simulink library "vehdynlibtirecommon_TUM"  (R2018b)
settings: Solver=ode45  StartTime=0.0  StopTime=10.0  RelTol=1e-3  EnableMultiTasking=on
undefined symbols (not defined in the file): br, drum_a, drum_abore, drum_c, drum_r, drum_theta1, drum_theta2, g, IYY, mu_kinetic, mu_static, omegao, T_RelaxationMy, tireStruct, UNLOADED_RADIUS, zdoto, zo
libraries: autolibsharedcommon x2, autolibutils x1
Description:
  | Automotive Blockset Library: Components used in the Tire Dynamics Library
settings Model: ModifiedByFormat=The MathWorks, Inc.  Creator=The MathWorks, Inc.  LastModifiedBy=The MathWorks, Inc.
settings SolverCC: MinimalZcImpactIntegration=on
settings DataIOCC: LimitDataPoints=on  SaveFormat=Array
settings OptimizationCC: LifeSpan=inf
settings DebuggingCC: AllowSymbolicDim=off  LibraryContextMissingDiagnostic=none  SFUnexpectedBacktrackingDiag=warning  SFNoUnconditionalDefaultTransitionDiag=warning  SFExecutionAtInitializationDiag=none
settings HardwareCC: ProdBitPerPointer=32  ProdBitPerSizeT=32  ProdBitPerPtrDiffT=32  ProdLargestAtomicFloat=None  ProdIntDivRoundTo=Undefined  ProdEndianess=Unspecified  ProdWordSize=32  ProdHWDeviceType=32-bit Generic
settings ModelReferenceCC: PropagateSignalLabelsOutOfModel=off
settings SFSimCC: SimUseLocalCustomCode=off
settings RTWCC: RTWUseLocalCustomCode=off
settings CodeAppCC: StateflowObjectComments=on
settings GRTTargetCC: TargetLangStandard=C89/C90 (ANSI)  GeneratePreprocessorConditionals=Disable all
settings ConfigComp: CovMetricSettings=dw  CovHtmlReporting=on  CovSaveCumulativeToWorkspaceVar=on  CovSaveSingleToWorkspaceVar=on  CovShowResultsExplorer=off  CovExternalEMLEnable=off

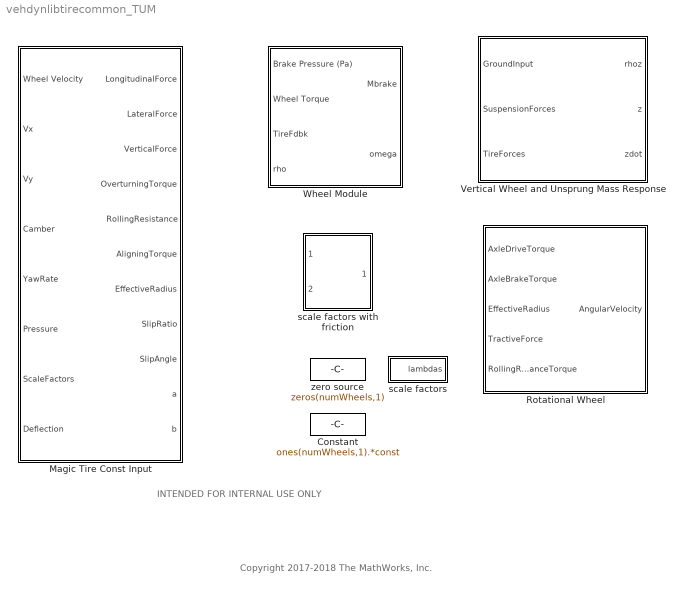
== system vehdynlibtirecommon_TUM ==
  note: INTENDED FOR INTERNAL USE ONLY
  note: Copyright 2017-2018 The MathWorks, Inc.
  Constant : Constant  Value=ones(numWheels,1).*const  mask{const=220000, numWheels=1}
      mask prompts: const "Constant Value"; numWheels "Number of wheels"
  Magic Tire Const Input : Subsystem
  Rotational Wheel : Subsystem  mask{Iyy=tireStruct(:).IYY, rhodot_o=omegao, br=br}
      mask prompts: Iyy "Wheel inertia [kg*m^2]"; rhodot_o "Initial wheel velocity [rad/s]"; br "Rotational damping [N*m*s/rad]"
  Vertical Wheel and Unsprung Mass Response : Subsystem  mask{m=tireStruct(:).MASS, bz=vertcat(tireStruct(:).VERTICAL_DAMPING), zo=zo, zdoto=zdoto, g=g, ReMax=.15}
      mask prompts: m "Unsprung mass [m]"; bz "Vertical damping [N*m/s]"; zo "Initial deflection [m]"; zdoto "Initial velocity [m/s]"; g "Gravitational acceleration [m/s^2]"; ReMax "Maximum unloaded radius [m]:"
  Wheel Module : Subsystem
  scale factors : Subsystem  mask{numWheels=1}
      mask prompts: numWheels "Number of wheels"
  scale factors with friction : Subsystem  mask{numWheels=1}
      mask prompts: numWheels "Number of wheels"
  zero source : Constant  Value=zeros(numWheels,1)  mask{numWheels=1}
      mask prompts: numWheels "Number of wheels"

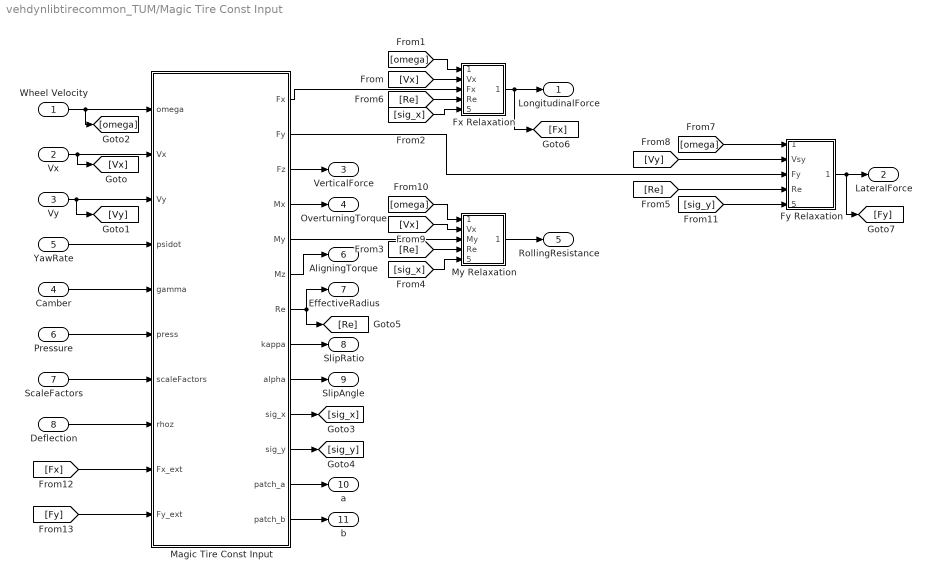
== system vehdynlibtirecommon_TUM/Magic Tire Const Input ==
  Wheel Velocity : Inport
  Vx : Inport  Port=2
  Vy : Inport  Port=3
  Camber : Inport  Port=4
  YawRate : Inport  Port=5
  Pressure : Inport  Port=6
  ScaleFactors : Inport  Port=7
  Deflection : Inport  Port=8
  Fx Relaxation : Subsystem
  Fy Relaxation : Subsystem
  Magic Tire Const Input : MATLAB Function
  My Relaxation : Subsystem
  LongitudinalForce : Outport
  LateralForce : Outport  Port=2
  VerticalForce : Outport  Port=3
  OverturningTorque : Outport  Port=4
  RollingResistance : Outport  Port=5
  AligningTorque : Outport  Port=6
  EffectiveRadius : Outport  Port=7
  SlipRatio : Outport  Port=8
  SlipAngle : Outport  Port=9
  a : Outport  Port=10
  b : Outport  Port=11
  wires:
  Magic Tire Const Input/3(Fz) -> VerticalForce/1
  Wheel Velocity/1 -> Magic Tire Const Input/1(omega), [omega]
  YawRate/1 -> Magic Tire Const Input/4(psidot)
  Camber/1 -> Magic Tire Const Input/5(gamma)
  Pressure/1 -> Magic Tire Const Input/6(press)
  ScaleFactors/1 -> Magic Tire Const Input/7(scaleFactors)
  Deflection/1 -> Magic Tire Const Input/8(rhoz)
  Magic Tire Const Input/4(Mx) -> OverturningTorque/1
  Magic Tire Const Input/6(Mz) -> AligningTorque/1
  Magic Tire Const Input/8(kappa) -> SlipRatio/1
  Magic Tire Const Input/9(alpha) -> SlipAngle/1
  Magic Tire Const Input/2(Fy) -> Fy Relaxation/3(Fy)
  Magic Tire Const Input/7(Re) -> [Re], EffectiveRadius/1
  Fx Relaxation/1(Out1) -> LongitudinalForce/1, [Fx]
  My Relaxation/1(Out1) -> RollingResistance/1
  Vx/1 -> [Vx], Magic Tire Const Input/2(Vx)
  Vy/1 -> [Vy], Magic Tire Const Input/3(Vy)
  Magic Tire Const Input/5(My) -> My Relaxation/3(My)
  Magic Tire Const Input/13(patch_b) -> b/1
  Magic Tire Const Input/12(patch_a) -> a/1
  Fy Relaxation/1(Out1) -> [Fy], LateralForce/1
  [Vx] -> Fx Relaxation/2(Vx)
  [omega] -> Fx Relaxation/1(omega)
  Magic Tire Const Input/10(sig_x) -> [sig_x]
  Magic Tire Const Input/11(sig_y) -> [sig_y]
  [sig_x] -> Fx Relaxation/5(sig_x)
  [Re] -> My Relaxation/4(Re)
  [sig_x] -> My Relaxation/5(sig_x)
  [Re] -> Fy Relaxation/4(Re)
  [Re] -> Fx Relaxation/4(Re)
  [omega] -> Fy Relaxation/1(omega)
  [Vy] -> Fy Relaxation/2(Vsy)
  [Vx] -> My Relaxation/2(Vx)
  [omega] -> My Relaxation/1(omega)
  [sig_y] -> Fy Relaxation/5(sig_y)
  Magic Tire Const Input/1(Fx) -> Fx Relaxation/3(Fx)
  [Fx] -> Magic Tire Const Input/9(Fx_ext)
  [Fy] -> Magic Tire Const Input/10(Fy_ext)

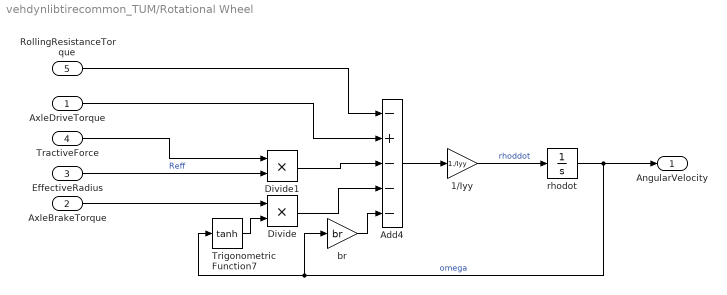
== system vehdynlibtirecommon_TUM/Rotational Wheel ==
  AxleDriveTorque : Inport
  AxleBrakeTorque : Inport  Port=2
  EffectiveRadius : Inport  Port=3
  TractiveForce : Inport  Port=4
  RollingResistanceTorque : Inport  Port=5
  1/Iyy : Gain  Gain=1./Iyy
  Add4 : Sum  Inputs=-+---
  Divide : Product  Inputs=**
  Divide1 : Product  Inputs=**
  Trigonometric Function7 : Trigonometry  Operator=tanh
  br : Gain  Gain=br
  "rhodot " : Integrator  InitialCondition=rhodot_o
  AngularVelocity : Outport
  wires:
  RollingResistanceTorque/1 -> Add4/1
  br/1 -> Add4/5
  AxleBrakeTorque/1 -> Divide/1
  AxleDriveTorque/1 -> Add4/2
  "rhodot "/1 -> AngularVelocity/1, Trigonometric Function7/1, br/1  "omega"
  Divide1/1 -> Add4/3
  EffectiveRadius/1 -> Divide1/2  "Reff"
  TractiveForce/1 -> Divide1/1
  Trigonometric Function7/1 -> Divide/2
  Divide/1 -> Add4/4
  Add4/1 -> 1/Iyy/1
  1/Iyy/1 -> "rhodot "/1  "rhoddot"

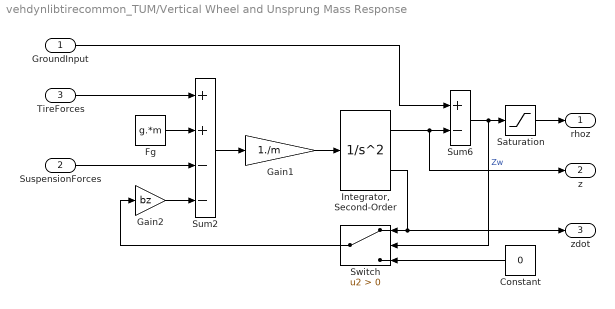
== system vehdynlibtirecommon_TUM/Vertical Wheel and Unsprung Mass Response ==
  GroundInput : Inport
  SuspensionForces : Inport  Port=2
  TireForces : Inport  Port=3
  Constant : Constant  Value=0
  Fg : Constant  Value=g.*m
  Gain1 : Gain  Gain=1./m  SaturateOnIntegerOverflow=on  OutDataTypeStr=Inherit: Same as input  ParamDataTypeStr=Inherit: Same as input
  Gain2 : Gain  Gain=bz  SaturateOnIntegerOverflow=on  OutDataTypeStr=Inherit: Same as input  ParamDataTypeStr=Inherit: Same as input
  "Integrator, Second-Order" : SecondOrderIntegrator  ICX=-zo  UpperLimitX=ReMax  LowerLimitX=0  ICDXDT=zdoto
  Saturation : Saturate  UpperLimit=inf  LowerLimit=0  ZeroCross=off
  Sum2 : Sum  Inputs=++--  SaturateOnIntegerOverflow=on  InputSameDT=on  OutDataTypeStr=Inherit: Same as first input
  Sum6 : Sum  Inputs=+-  SaturateOnIntegerOverflow=on  InputSameDT=on  OutDataTypeStr=Inherit: Same as first input
  Switch : Switch  Criteria=u2 > Threshold  ZeroCross=off
  rhoz : Outport
  z : Outport  Port=2
  zdot : Outport  Port=3
  wires:
  "Integrator, Second-Order"/2 -> zdot/1, Switch/1
  Gain2/1 -> Sum2/4
  Fg/1 -> Sum2/2
  Saturation/1 -> rhoz/1
  GroundInput/1 -> Sum6/1
  "Integrator, Second-Order"/1 -> Sum6/2, z/1  "Zw"
  Gain1/1 -> "Integrator, Second-Order"/1
  Sum2/1 -> Gain1/1
  SuspensionForces/1 -> Sum2/3
  TireForces/1 -> Sum2/1
  Sum6/1 -> Switch/2, Saturation/1
  Switch/1 -> Gain2/1
  Constant/1 -> Switch/3

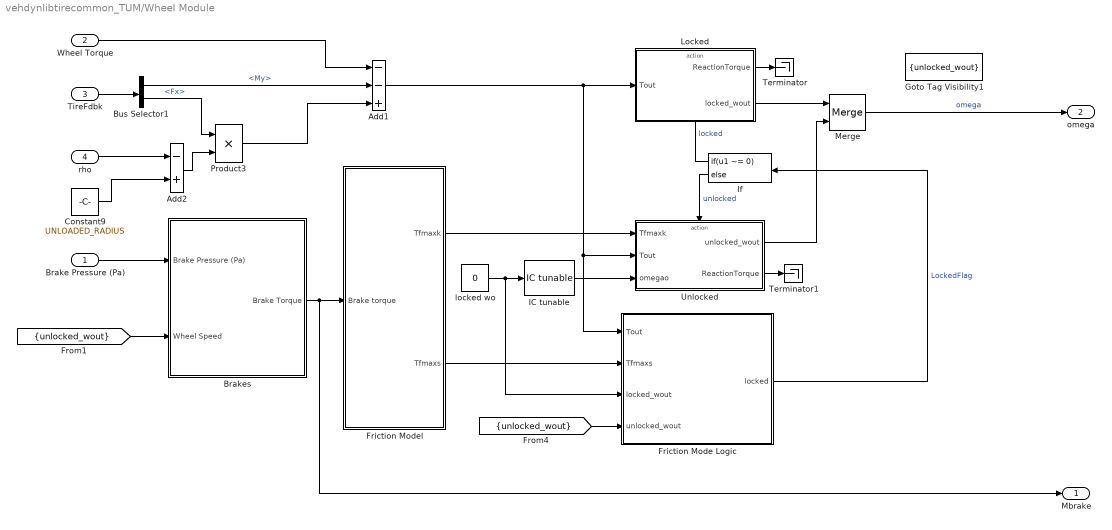
== system vehdynlibtirecommon_TUM/Wheel Module ==
  Brake Pressure (Pa) : Inport
  Wheel Torque : Inport  Port=2
  TireFdbk : Inport  Port=3
  rho : Inport  Port=4
  Add1 : Sum  Inputs=--+
  Add2 : Sum  Inputs=-+
  Brakes : Subsystem  VariantControlMode=Label  Variant=on  LabelModeActiveChoice=Disk
  Bus Selector1 : BusSelector  OutputSignals=My,Fx
  Constant9 : Constant  Value=UNLOADED_RADIUS
  Friction Model : Subsystem
  Friction Mode Logic : Subsystem
      mask Display: plot([-3 1 1 3 -1 -1],[-1 -1 1 1 1 -1],-4,-5,4,5)
  Goto Tag Visibility1 : GotoTagVisibility  GotoTag=unlocked_wout
  IC tunable : autolibutils/IC tunable  IC=omegao  aMode=2
      settings: SourceProductName=Powertrain Blockset  SourceProductBaseCode=PW
  If : If  IfExpression=u1 ~= 0
  Locked : Subsystem  TreatAsAtomicUnit=on
      mask Display: plot(-1,-6,6,12,[0 3],[3 3],[3 1 1 3], [1 1 5 5],[2 4 4 2],[4 4 2 2],[4 5],[3 3])
  Merge : Merge
  Product3 : Product  Inputs=**
  Terminator : Terminator
  Terminator1 : Terminator
  Unlocked : Subsystem  TreatAsAtomicUnit=on
      mask Display: plot(-1,-2,6,8,[0 3],[3 3],[3 1 1 3], [1 1 5 5],[2 4 4 2],[4 4 2 2],[4 5],[3 3])
  locked wo : Constant  Value=0
  Mbrake : Outport
  omega : Outport  Port=2
  wires:
  TireFdbk/1 -> Bus Selector1/1
  Bus Selector1/1 -> Add1/2  "<My>"
  Bus Selector1/2 -> Product3/1  "<Fx>"
  Merge/1 -> omega/1  "omega"
  Locked/2(locked_wout) -> Merge/1
  locked wo/1 -> Friction Mode Logic/3(locked_wout), IC tunable/1
  IC tunable/1 -> Unlocked/3(omegao)
  Brakes/1(Brake Torque) -> Friction Model/1(Brake torque), Mbrake/1
  [unlocked_wout] -> Brakes/2(Wheel Speed)
  Brake Pressure (Pa)/1 -> Brakes/1(Brake Pressure (Pa))
  Unlocked/2(ReactionTorque) -> Terminator1/1
  Locked/1(ReactionTorque) -> Terminator/1
  Add1/1 -> Locked/1(Tout), Unlocked/2(Tout), Friction Mode Logic/1(Tout)
  Wheel Torque/1 -> Add1/1
  Friction Model/2(Tfmaxs) -> Friction Mode Logic/2(Tfmaxs)
  Friction Model/1(Tfmaxk) -> Unlocked/1(Tfmaxk)
  [unlocked_wout] -> Friction Mode Logic/4(unlocked_wout)
  If/2 -> Unlocked/Action  "unlocked"
  If/1 -> Locked/Action  "locked"
  Friction Mode Logic/1(locked) -> If/1  "LockedFlag"
  Unlocked/1(unlocked_wout) -> Merge/2
  rho/1 -> Add2/1
  Constant9/1 -> Add2/2
  Add2/1 -> Product3/2
  Product3/1 -> Add1/3

== system vehdynlibtirecommon_TUM/scale factors ==
  ones2 : Constant  Value=[ones(3,numWheels);zeros(1,numWheels);ones(23,numWheels)]
  lambdas : Outport
  wires:
  ones2/1 -> lambdas/1

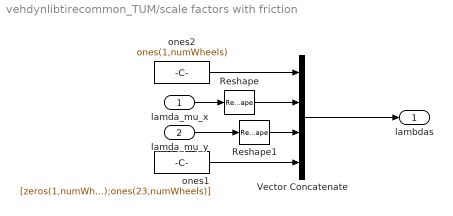
== system vehdynlibtirecommon_TUM/scale factors with friction ==
  lamda_mu_x : Inport
  lamda_mu_y : Inport  Port=2
  Reshape : Reshape  OutputDimensionality=Row vector (2-D)  OutputDimensions=[1,numWheels]
  Reshape1 : Reshape  OutputDimensionality=Row vector (2-D)  OutputDimensions=[1,numWheels]
  Vector Concatenate : Concatenate  NumInputs=4  Mode=Multidimensional array
  ones1 : Constant  Value=[zeros(1,numWheels);ones(23,numWheels)]  VectorParams1D=off
  ones2 : Constant  Value=ones(1,numWheels)  VectorParams1D=off
  lambdas : Outport
  wires:
  Reshape1/1 -> Vector Concatenate/3
  Reshape/1 -> Vector Concatenate/2
  lamda_mu_y/1 -> Reshape1/1
  lamda_mu_x/1 -> Reshape/1
  ones1/1 -> Vector Concatenate/4
  Vector Concatenate/1 -> lambdas/1
  ones2/1 -> Vector Concatenate/1

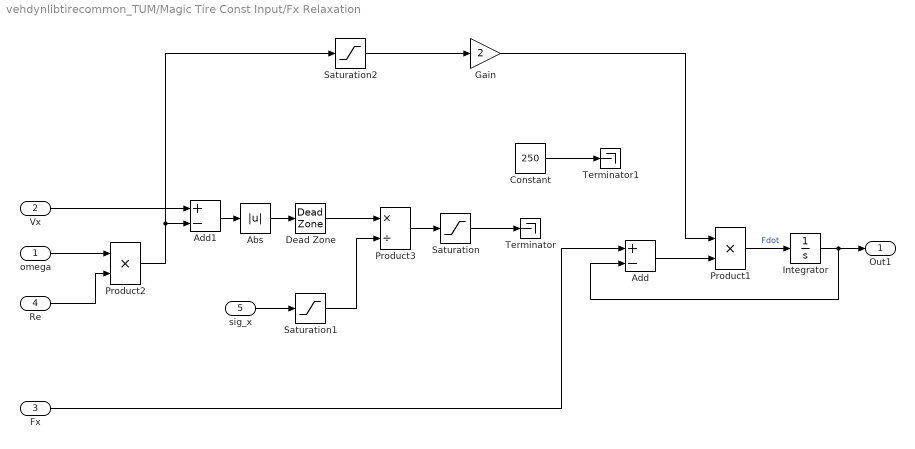
== system vehdynlibtirecommon_TUM/Magic Tire Const Input/Fx Relaxation ==
  omega : Inport
  Vx : Inport  Port=2
  Fx : Inport  Port=3
  Re : Inport  Port=4
  sig_x : Inport  Port=5
  Abs : Abs  ZeroCross=off
  Add : Sum  Inputs=+-
  Add1 : Sum  Inputs=+-
  Constant : Constant  Value=250
  Dead Zone : DeadZone  LowerValue=0  UpperValue=VXLOW  ZeroCross=off  SaturateOnIntegerOverflow=on
  Gain : Gain  Gain=2
  Integrator : Integrator  UpperSaturationLimit=10e3  LowerSaturationLimit=-10e3  AbsoluteTolerance=1e-3  ZeroCross=off
  Product1 : Product  Inputs=**
  Product2 : Product  Inputs=**
  Product3 : Product  Inputs=*/
  Saturation : Saturate  UpperLimit=400*pi*2  LowerLimit=2*pi  ZeroCross=off
  Saturation1 : Saturate  UpperLimit=10  LowerLimit=.01  ZeroCross=off
  Saturation2 : Saturate  UpperLimit=100  LowerLimit=10
  Terminator : Terminator
  Terminator1 : Terminator
  Out1 : Outport  PortDimensions=1
  wires:
  Abs/1 -> Dead Zone/1
  Vx/1 -> Add1/1
  Product3/1 -> Saturation/1
  Re/1 -> Product2/2
  omega/1 -> Product2/1
  Fx/1 -> Add/1
  Integrator/1 -> Add/2, Out1/1
  Product1/1 -> Integrator/1  "Fdot"
  Add/1 -> Product1/2
  Add1/1 -> Abs/1
  Saturation/1 -> Terminator/1
  Dead Zone/1 -> Product3/1
  sig_x/1 -> Saturation1/1
  Saturation1/1 -> Product3/2
  Gain/1 -> Product1/1
  Saturation2/1 -> Gain/1
  Product2/1 -> Saturation2/1, Add1/2
  Constant/1 -> Terminator1/1

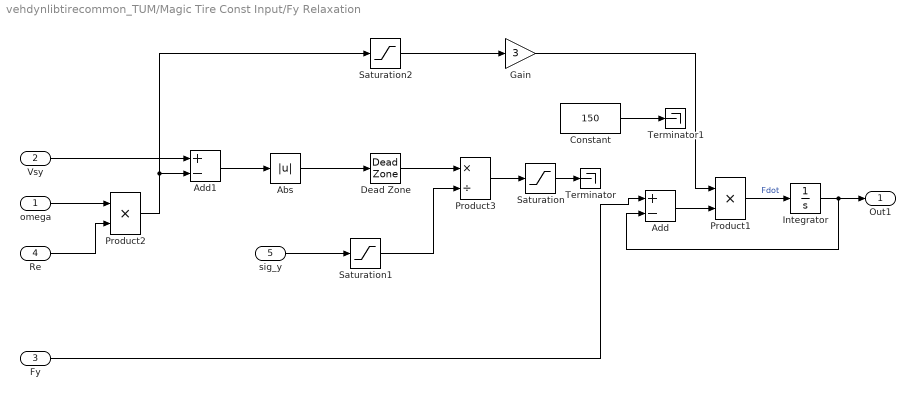
== system vehdynlibtirecommon_TUM/Magic Tire Const Input/Fy Relaxation ==
  omega : Inport
  Vsy : Inport  Port=2
  Fy : Inport  Port=3
  Re : Inport  Port=4
  sig_y : Inport  Port=5
  Abs : Abs  ZeroCross=off
  Add : Sum  Inputs=+-
  Add1 : Sum  Inputs=+-
  Constant : Constant  Value=150
  Dead Zone : DeadZone  LowerValue=0  UpperValue=VXLOW  ZeroCross=off  SaturateOnIntegerOverflow=on
  Gain : Gain  Gain=3
  Integrator : Integrator  UpperSaturationLimit=10e3  LowerSaturationLimit=-10e3  AbsoluteTolerance=1e-3  ZeroCross=off
  Product1 : Product  Inputs=**
  Product2 : Product  Inputs=**
  Product3 : Product  Inputs=*/
  Saturation : Saturate  UpperLimit=400*pi  LowerLimit=2*pi  ZeroCross=off
  Saturation1 : Saturate  UpperLimit=10  LowerLimit=.01  ZeroCross=off
  Saturation2 : Saturate  UpperLimit=100  LowerLimit=1
  Terminator : Terminator
  Terminator1 : Terminator
  Out1 : Outport  PortDimensions=1
  wires:
  Add/1 -> Product1/2
  Product1/1 -> Integrator/1  "Fdot"
  Integrator/1 -> Out1/1, Add/2
  Fy/1 -> Add/1
  omega/1 -> Product2/1
  Re/1 -> Product2/2
  Product3/1 -> Saturation/1
  Vsy/1 -> Add1/1
  Product2/1 -> Saturation2/1, Add1/2
  Abs/1 -> Dead Zone/1
  Dead Zone/1 -> Product3/1
  Add1/1 -> Abs/1
  sig_y/1 -> Saturation1/1
  Saturation1/1 -> Product3/2
  Saturation/1 -> Terminator/1
  Saturation2/1 -> Gain/1
  Gain/1 -> Product1/1
  Constant/1 -> Terminator1/1

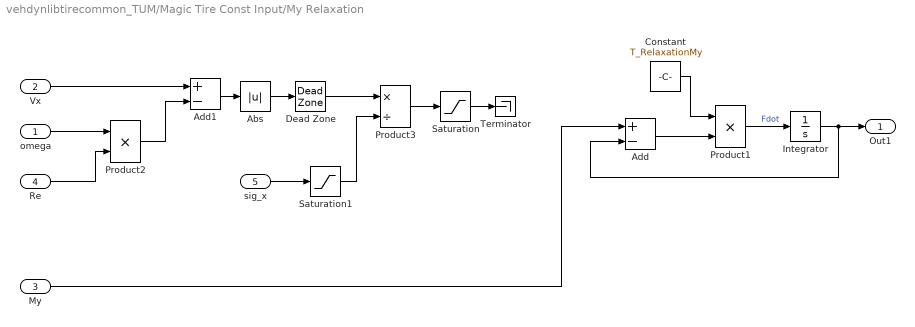
== system vehdynlibtirecommon_TUM/Magic Tire Const Input/My Relaxation ==
  omega : Inport
  Vx : Inport  Port=2
  My : Inport  Port=3
  Re : Inport  Port=4
  sig_x : Inport  Port=5
  Abs : Abs  ZeroCross=off
  Add : Sum  Inputs=+-
  Add1 : Sum  Inputs=+-
  Constant : Constant  Value=T_RelaxationMy
  Dead Zone : DeadZone  LowerValue=0  UpperValue=VXLOW  ZeroCross=off  SaturateOnIntegerOverflow=on
  Integrator : Integrator  UpperSaturationLimit=10e3  LowerSaturationLimit=-10e3  AbsoluteTolerance=1e-3  ZeroCross=off
  Product1 : Product  Inputs=**
  Product2 : Product  Inputs=**
  Product3 : Product  Inputs=*/
  Saturation : Saturate  UpperLimit=400*pi*2  LowerLimit=2*pi  ZeroCross=off
  Saturation1 : Saturate  UpperLimit=10  LowerLimit=.01  ZeroCross=off
  Terminator : Terminator
  Out1 : Outport  PortDimensions=1
  wires:
  Dead Zone/1 -> Product3/1
  Add1/1 -> Abs/1
  Add/1 -> Product1/2
  Product1/1 -> Integrator/1  "Fdot"
  Integrator/1 -> Out1/1, Add/2
  My/1 -> Add/1
  omega/1 -> Product2/1
  Re/1 -> Product2/2
  Product3/1 -> Saturation/1
  Vx/1 -> Add1/1
  Product2/1 -> Add1/2
  Abs/1 -> Dead Zone/1
  sig_x/1 -> Saturation1/1
  Saturation1/1 -> Product3/2
  Saturation/1 -> Terminator/1
  Constant/1 -> Product1/1

== system vehdynlibtirecommon_TUM/Wheel Module/Brakes ==
  note: 1) Add Subsystem or Model blocks as valid variant choices.
      | 2) You cannot connect blocks at this level. At simulation, connectivity is automatically
      | determined, based on the active variant and port name matching.
  Brake Pressure (Pa) : Inport
  Wheel Speed : Inport  Port=2
  Disk Brake : Subsystem  VariantControl=Disk
  Drum Brake : Subsystem  VariantControl=Drum
  Mapped Brake : Subsystem  VariantControl=Mapped
  No Brake : Subsystem  VariantControl=None
  Brake Torque : Outport

== system vehdynlibtirecommon_TUM/Wheel Module/Friction Model ==
  Brake torque : Inport
  Ratio of static to kinetic : Gain  Gain=mu_static/mu_kinetic  SaturateOnIntegerOverflow=on  OutDataTypeStr=Inherit: Same as input  ParamDataTypeStr=Inherit: Same as input
  Tfmaxk : Outport  InitialOutput=0
  Tfmaxs : Outport  Port=2  InitialOutput=0
  wires:
  Ratio of static to kinetic/1 -> Tfmaxs/1
  Brake torque/1 -> Ratio of static to kinetic/1, Tfmaxk/1

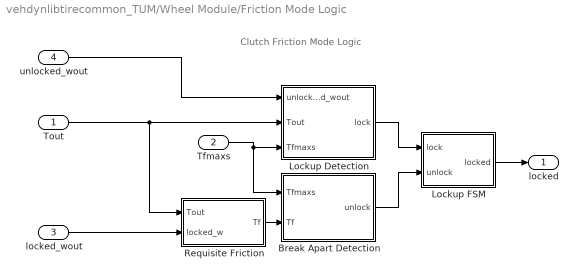
== system vehdynlibtirecommon_TUM/Wheel Module/Friction Mode Logic ==
  note: Clutch Friction Mode Logic
  Tout : Inport
  Tfmaxs : Inport  Port=2
  locked_wout : Inport  Port=3
  unlocked_wout : Inport  Port=4
  Break Apart Detection : Subsystem
  Lockup Detection : Subsystem
  Lockup FSM : Subsystem
  Requisite Friction : Subsystem
  locked : Outport  InitialOutput=0
  wires:
  Tout/1 -> Requisite Friction/1(Tout), Lockup Detection/2(Tout)
  unlocked_wout/1 -> Lockup Detection/1(unlocked_wout)
  locked_wout/1 -> Requisite Friction/2(locked_w)
  Lockup FSM/1(locked) -> locked/1
  Lockup Detection/1(lock) -> Lockup FSM/1(lock)
  Break Apart Detection/1(unlock) -> Lockup FSM/2(unlock)
  Requisite Friction/1(Tf) -> Break Apart Detection/2(Tf)
  Tfmaxs/1 -> Lockup Detection/3(Tfmaxs), Break Apart Detection/1(Tfmaxs)

== system vehdynlibtirecommon_TUM/Wheel Module/Locked ==
  Tout : Inport
  Action : ActionPort  InitializeStates=reset
  Unary Minus : UnaryMinus
  locked : Constant  Value=0
  ReactionTorque : Outport  InitialOutput=0
  locked_wout : Outport  Port=2  InitialOutput=0
  wires:
  locked/1 -> locked_wout/1
  Tout/1 -> Unary Minus/1
  Unary Minus/1 -> ReactionTorque/1

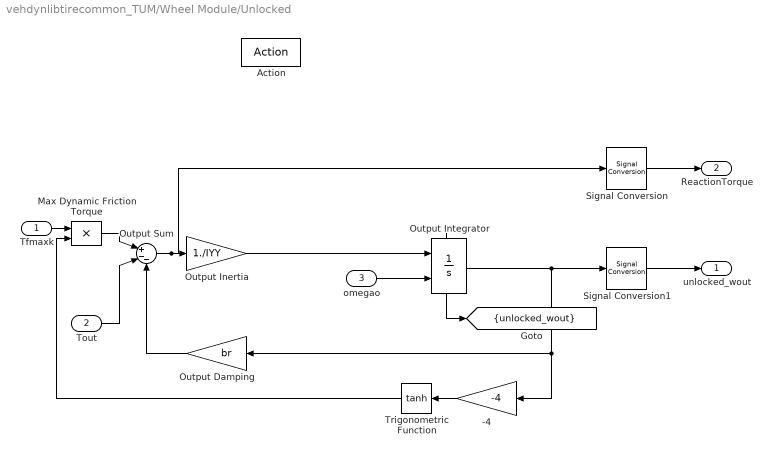
== system vehdynlibtirecommon_TUM/Wheel Module/Unlocked ==
  Tfmaxk : Inport
  Tout : Inport  Port=2
  omegao : Inport  Port=3
  Action : ActionPort  InitializeStates=reset
  -4 : Gain  Gain=-4  SaturateOnIntegerOverflow=on  OutDataTypeStr=Inherit: Same as input  ParamDataTypeStr=Inherit: Same as input
  Max Dynamic Friction Torque : Product  SaturateOnIntegerOverflow=on  RndMeth=Zero  InputSameDT=on  OutDataTypeStr=Inherit: Same as first input
  Output Inertia : Gain  Gain=1./IYY  SaturateOnIntegerOverflow=on  OutDataTypeStr=Inherit: Same as input  ParamDataTypeStr=Inherit: Same as input
  Output Integrator : Integrator  InitialConditionSource=external  ShowStatePort=on
  Output Damping : Gain  Gain=br  SaturateOnIntegerOverflow=on  OutDataTypeStr=Inherit: Same as input  ParamDataTypeStr=Inherit: Same as input
  Output Sum : Sum  Inputs=|+--  SaturateOnIntegerOverflow=on  InputSameDT=on  OutDataTypeStr=Inherit: Same as first input
  Signal Conversion : SignalConversion  OverrideOpt=off
  Signal Conversion1 : SignalConversion  OverrideOpt=off
  Trigonometric Function : Trigonometry  Operator=tanh
  unlocked_wout : Outport  InitialOutput=0
  ReactionTorque : Outport  Port=2  InitialOutput=0
  tag scope: unlocked_wout=scoped
  wires:
  Signal Conversion1/1 -> unlocked_wout/1
  omegao/1 -> Output Integrator/2
  -4/1 -> Trigonometric Function/1
  Tout/1 -> Output Sum/2
  Output Integrator/State -> [unlocked_wout]
  Output Integrator/1 -> Output Damping/1, -4/1, Signal Conversion1/1
  Output Inertia/1 -> Output Integrator/1
  Trigonometric Function/1 -> Max Dynamic Friction Torque/2
  Tfmaxk/1 -> Max Dynamic Friction Torque/1
  Max Dynamic Friction Torque/1 -> Output Sum/1
  Output Damping/1 -> Output Sum/3
  Output Sum/1 -> Signal Conversion/1, Output Inertia/1
  Signal Conversion/1 -> ReactionTorque/1

== system vehdynlibtirecommon_TUM/Wheel Module/Brakes/Disk Brake ==
  Brake Pressure (Pa) : Inport
  Wheel Speed : Inport  Port=2
  Disk Brake : autolibsharedcommon/Disk Brake  disk_abore=disk_abore  num_pads=num_pads  Rm=Rm  mu_kinetic=mu_kinetic
      settings: SourceProductName=Powertrain Blockset  SourceProductBaseCode=PW
  Brake Torque : Outport
  wires:
  Brake Pressure (Pa)/1 -> Disk Brake/1
  Wheel Speed/1 -> Disk Brake/2
  Disk Brake/1 -> Brake Torque/1

== system vehdynlibtirecommon_TUM/Wheel Module/Brakes/Drum Brake ==
  Brake Pressure (Pa) : Inport
  Wheel Speed : Inport  Port=2
  Drum Brake : Subsystem  mask{drum_abore=drum_abore, mu_kinetic=mu_kinetic, drum_a=drum_a, drum_c=drum_c, drum_r=drum_r, drum_theta1=drum_theta1, drum_theta2=drum_theta2}
      mask prompts: drum_abore "Drum brake actuator bore, drum_abore [m]:"; mu_kinetic "Kinetic friction coefficient, mu_kinetic [-]:"; drum_a "Shoe pin to drum center distance, drum_a [m]:"; drum_c "Shoe pin center to force application point distance, drum_c [m]:"; drum_r "Drum internal radius, drum_r [m]:"; drum_theta1 "Shoe pin to pad start angle, drum_theta1 [deg]:"; drum_theta2 "Shoe pin to pad end angle, drum_theta2 [deg]:"
      mask help: Implements a drum brake pressure to torque transformation model based on the drum and shoe geometry parameters provided by the user.
  Brake Torque : Outport
  wires:
  Drum Brake/1(Brake Torque) -> Brake Torque/1
  Wheel Speed/1 -> Drum Brake/2(Wheel angular velocity)
  Brake Pressure (Pa)/1 -> Drum Brake/1(Brake Pressure)

== system vehdynlibtirecommon_TUM/Wheel Module/Brakes/Mapped Brake ==
  Brake Pressure (Pa) : Inport
  Wheel Speed : Inport  Port=2
  Mapped Brake : autolibsharedcommon/Mapped Brake  brake_p_bpt=brake_p_bpt  brake_n_bpt=brake_n_bpt  f_brake_t=f_brake_t
      settings: SourceProductName=Powertrain Blockset  SourceProductBaseCode=PW
  Brake Torque : Outport
  wires:
  Wheel Speed/1 -> Mapped Brake/2
  Mapped Brake/1 -> Brake Torque/1
  Brake Pressure (Pa)/1 -> Mapped Brake/1

== system vehdynlibtirecommon_TUM/Wheel Module/Brakes/No Brake ==
  Brake Pressure (Pa) : Inport
  Wheel Speed : Inport  Port=2
  Ground : Ground
  Terminator : Terminator
  Terminator1 : Terminator
  Brake Torque : Outport
  wires:
  Brake Pressure (Pa)/1 -> Terminator/1
  Ground/1 -> Brake Torque/1
  Wheel Speed/1 -> Terminator1/1

== system vehdynlibtirecommon_TUM/Wheel Module/Friction Mode Logic/Break Apart Detection ==
  Tfmaxs : Inport
  Tf : Inport  Port=2
  Abs : Abs  ZeroCross=off  SaturateOnIntegerOverflow=on
  Relational Operator : RelationalOperator  OutDataTypeStr=boolean  ZeroCross=off  RndMeth=Nearest  InputSameDT=on
  unlock : Outport  InitialOutput=0
  wires:
  Tfmaxs/1 -> Relational Operator/2
  Abs/1 -> Relational Operator/1
  Relational Operator/1 -> unlock/1
  Tf/1 -> Abs/1

== system vehdynlibtirecommon_TUM/Wheel Module/Friction Mode Logic/Lockup Detection ==
  unlocked_wout : Inport
  Tout : Inport  Port=2
  Tfmaxs : Inport  Port=3
  Friction Calc : Subsystem
  Logic : Logic  IconShape=distinctive  OutDataTypeStr=boolean
  Required Friction for Lockup : Subsystem
  Velocities Match : HitCross  ZeroCross=off
  lock : Outport  InitialOutput=0
  wires:
  unlocked_wout/1 -> Velocities Match/1
  Required Friction for Lockup/1(okay) -> Logic/2
  Logic/1 -> lock/1
  Velocities Match/1 -> Logic/1
  Tfmaxs/1 -> Required Friction for Lockup/2(Max Friction Torque)
  Friction Calc/1(Friction Torque) -> Required Friction for Lockup/1(Friction Torque)
  Tout/1 -> Friction Calc/1(Tout)

== system vehdynlibtirecommon_TUM/Wheel Module/Friction Mode Logic/Lockup FSM ==
  lock : Inport
  unlock : Inport  Port=2
  Combinatorial Logic : CombinatorialLogic  TruthTable=[0;1;0;0;1;1;1;0]
  Memory : Memory
  Mux : Mux  Inputs=3
  locked : Outport  InitialOutput=0
  wires:
  Mux/1 -> Combinatorial Logic/1
  lock/1 -> Mux/1
  unlock/1 -> Mux/2
  Combinatorial Logic/1 -> Memory/1, locked/1
  Memory/1 -> Mux/3

== system vehdynlibtirecommon_TUM/Wheel Module/Friction Mode Logic/Requisite Friction ==
  Tout : Inport
  locked_w : Inport  Port=2
  Output Damping : Gain  Gain=br  SaturateOnIntegerOverflow=on  OutDataTypeStr=Inherit: Same as input  ParamDataTypeStr=Inherit: Same as input
  Sum1 : Sum  Inputs=|++  SaturateOnIntegerOverflow=on  InputSameDT=on  OutDataTypeStr=Inherit: Same as first input
  Sum2 : Sum  Inputs=|--  SaturateOnIntegerOverflow=on  InputSameDT=on  OutDataTypeStr=Inherit: Same as first input
  Tf : Outport  InitialOutput=0
  wires:
  Output Damping/1 -> Sum1/2, Sum2/2
  locked_w/1 -> Output Damping/1
  Tout/1 -> Sum2/1
  Sum2/1 -> Sum1/1
  Sum1/1 -> Tf/1

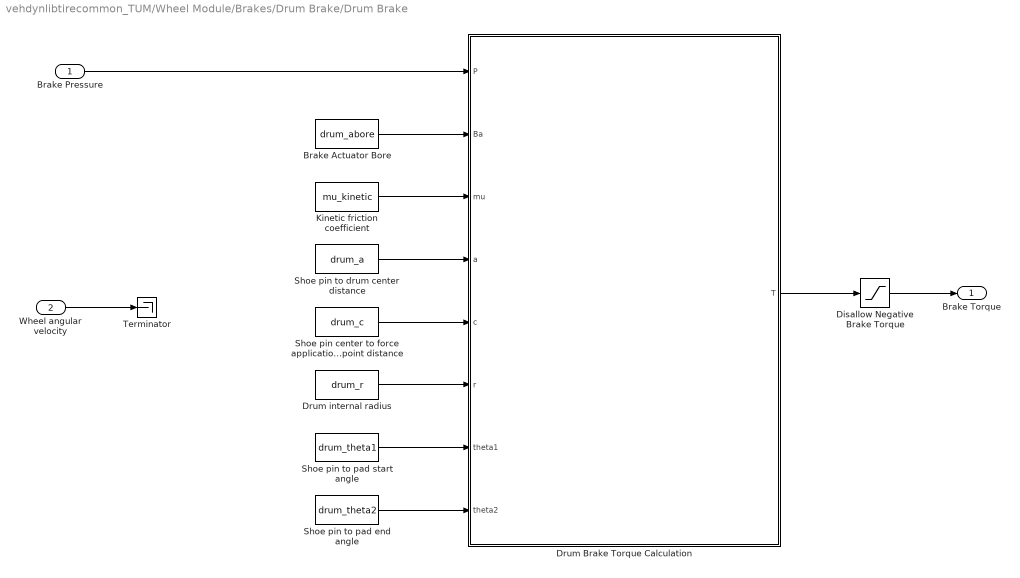
== system vehdynlibtirecommon_TUM/Wheel Module/Brakes/Drum Brake/Drum Brake ==
  Brake Pressure : Inport
  Wheel angular velocity : Inport  Port=2
  Brake Actuator Bore : Constant  Value=drum_abore
  Disallow Negative Brake Torque : Saturate  UpperLimit=inf  LowerLimit=eps
  Drum Brake Torque Calculation : MATLAB Function  TreatAsAtomicUnit=on
  Drum internal radius : Constant  Value=drum_r
  Kinetic friction coefficient : Constant  Value=mu_kinetic
  Shoe pin center to force application point distance : Constant  Value=drum_c
  Shoe pin to drum center distance : Constant  Value=drum_a
  Shoe pin to pad end angle : Constant  Value=drum_theta2
  Shoe pin to pad start angle : Constant  Value=drum_theta1
  Terminator : Terminator
  Brake Torque : Outport
  wires:
  Brake Pressure/1 -> Drum Brake Torque Calculation/1(P)
  Shoe pin to pad end angle/1 -> Drum Brake Torque Calculation/8(theta2)
  Shoe pin to pad start angle/1 -> Drum Brake Torque Calculation/7(theta1)
  Kinetic friction coefficient/1 -> Drum Brake Torque Calculation/3(mu)
  Drum Brake Torque Calculation/1(T) -> Disallow Negative Brake Torque/1
  Drum internal radius/1 -> Drum Brake Torque Calculation/6(r)
  Shoe pin center to force application point distance/1 -> Drum Brake Torque Calculation/5(c)
  Shoe pin to drum center distance/1 -> Drum Brake Torque Calculation/4(a)
  Wheel angular velocity/1 -> Terminator/1
  Brake Actuator Bore/1 -> Drum Brake Torque Calculation/2(Ba)
  Disallow Negative Brake Torque/1 -> Brake Torque/1

== system vehdynlibtirecommon_TUM/Wheel Module/Friction Mode Logic/Lockup Detection/Friction Calc ==
  Tout : Inport
  Unary Minus : UnaryMinus
  Friction Torque : Outport  InitialOutput=0
  wires:
  Tout/1 -> Unary Minus/1
  Unary Minus/1 -> Friction Torque/1

== system vehdynlibtirecommon_TUM/Wheel Module/Friction Mode Logic/Lockup Detection/Required Friction for Lockup ==
  Friction Torque : Inport
  Max Friction Torque : Inport  Port=2
  Abs : Abs  ZeroCross=off  SaturateOnIntegerOverflow=on
  Relational Operator : RelationalOperator  Operator=<=  OutDataTypeStr=boolean  ZeroCross=off  RndMeth=Nearest  InputSameDT=on
  okay : Outport  InitialOutput=0
  wires:
  Max Friction Torque/1 -> Relational Operator/2
  Abs/1 -> Relational Operator/1
  Relational Operator/1 -> okay/1
  Friction Torque/1 -> Abs/1

== matlab function vehdynlibtirecommon_TUM/Magic Tire Const Input/Magic Tire Const Input ==
  data: omega input; Vx input; Vy input; psidot input; gamma input; press input; scaleFactors input size=[27,1]; rhoz input; plySteer parameter; Fx output size=size(omega); Fy output double size=size(omega); Fz output size=size(omega); Mx output size=size(omega); My output size=size(omega); Mz output size=size(omega); Re output size=size(omega); kappa output size=size(omega); alpha output size=size(omega); sig_x output; sig_y output; PRESMAX parameter; PRESMIN parameter; FZMAX parameter; FZMIN parameter; VXLOW parameter; KPUMAX parameter; KPUMIN parameter; ALPMAX parameter; ALPMIN parameter; CAMMIN parameter; CAMMAX parameter; LONGVL parameter; UNLOADED_RADIUS parameter; NOMPRES parameter; FNOMIN parameter; VERTICAL_STIFFNESS parameter; DREFF parameter; BREFF parameter; FREFF parameter; Q_RE0 parameter; Q_V1 parameter; Q_V2 parameter; Q_FZ1 parameter; Q_FZ2 parameter; Q_FCX parameter; Q_FCY parameter; PFZ1 parameter; Q_FCY2 parameter; PCX1 parameter; PDX1 parameter; PDX2 parameter; PDX3 parameter; PEX1 parameter; PEX2 parameter; PEX3 parameter; PEX4 parameter; PKX1 parameter; PKX2 parameter; PKX3 parameter; PHX1 parameter; PHX2 parameter; PVX1 parameter; PVX2 parameter; PPX1 parameter; PPX2 parameter; PPX3 parameter; PPX4 parameter; RBX1 parameter; RBX2 parameter; RBX3 parameter; RCX1 parameter; REX1 parameter; REX2 parameter; RHX1 parameter; QSX1 parameter; QSX2 parameter; QSX3 parameter; QSX4 parameter; QSX5 parameter; QSX6 parameter; QSX7 parameter; QSX8 parameter; QSX9 parameter; QSX10 parameter; QSX11 parameter; PPMX1 parameter; PCY1 parameter; PDY1 parameter; PDY2 parameter; PDY3 parameter; PEY1 parameter; PEY2 parameter; PEY3 parameter; PEY4 parameter; PEY5 parameter; PKY1 parameter; PKY2 parameter; PKY3 parameter; PKY4 parameter; PKY5 parameter; PKY6 parameter; PKY7 parameter; PHY1 parameter; PHY2 parameter; PVY1 parameter; PVY2 parameter; PVY3 parameter; PVY4 parameter; PPY1 parameter; PPY2 parameter; PPY3 parameter; PPY4 parameter; PPY5 parameter; RBY1 parameter; RBY2 parameter; RBY3 parameter; RBY4 parameter; RCY1 parameter; REY1 parameter; REY2 parameter; RHY1 parameter; RHY2 parameter; RVY1 parameter; RVY2 parameter; RVY3 parameter; RVY4 parameter; RVY5 parameter; RVY6 parameter; QSY1 parameter; QSY2 parameter; QSY3 parameter; QSY4 parameter; QSY5 parameter; QSY6 parameter; QSY7 parameter; QSY8 parameter; QBZ1 parameter; QBZ2 parameter; QBZ3 parameter; QBZ4 parameter; QBZ5 parameter; QBZ6 parameter; QBZ9 parameter; QBZ10 parameter; QCZ1 parameter; QDZ1 parameter; QDZ2 parameter; QDZ3 parameter; QDZ4 parameter; QDZ6 parameter; QDZ7 parameter; QDZ8 parameter; QDZ9 parameter; QDZ10 parameter; QDZ11 parameter; QEZ1 parameter; QEZ2 parameter; QEZ3 parameter; QEZ4 parameter; QEZ5 parameter; QHZ1 parameter; QHZ2 parameter; QHZ3 parameter; QHZ4 parameter; PPZ1 parameter; PPZ2 parameter; SSZ1 parameter; SSZ2 parameter; SSZ3 parameter; SSZ4 parameter; PDXP1 parameter; PDXP2 parameter; PDXP3 parameter; PKYP1 parameter; PDYP1 parameter; PDYP2 parameter; PDYP3 parameter; PDYP4 parameter; PHYP1 parameter; PHYP2 parameter; PHYP3 parameter; PHYP4 parameter; PECP1 parameter; PECP2 parameter; QDTP1 parameter; QCRP1 parameter; QCRP2 parameter; QBRP1 parameter; QDRP1 parameter; QDRP2 parameter; WIDTH parameter; Q_RA1 parameter; Q_RA2 parameter; Q_RB1 parameter; Q_RB2 parameter; QSX12 parameter; QSX13 parameter; QSX14 parameter; patch_a output; patch_b output; Q_FZ3 parameter; LONGITUDINAL_STIFFNESS parameter; LATERAL_STIFFNESS parameter; PCFX1 parameter; PCFX2 parameter; PCFX3 parameter; PCFY1 parameter; PCFY2 parameter; PCFY3 parameter; Fx_ext input; Fy_ext input
function [Fx,Fy,Fz,Mx,My,Mz,Re,kappa,alpha,sig_x,sig_y,patch_a,patch_b] = magictire(omega,Vx,Vy,psidot,gamma,press,scaleFactors,rhoz,plySteer,...
PRESMAX,...
PRESMIN,...
FZMAX,...
FZMIN,...
VXLOW,...
KPUMAX,...
KPUMIN,...
ALPMAX,...
ALPMIN,...
CAMMIN,...
CAMMAX,...
LONGVL,...
UNLOADED_RADIUS,...
NOMPRES,...
FNOMIN,...
VERTICAL_STIFFNESS,...% vertical
DREFF,...
BREFF,...
FREFF,...
Q_RE0,...
Q_V1,...
Q_V2,...
Q_FZ1,...
Q_FZ2,...
Q_FCX,...
Q_FCY,...
PFZ1,...
Q_FCY2,...
PCX1,...% longitudinal
PDX1,...
PDX2,...
PDX3,...
PEX1,...
PEX2,...
PEX3,...
PEX4,...
PKX1,...
PKX2,...
PKX3,...
PHX1,...
PHX2,...
PVX1,...
PVX2,...
PPX1,...
PPX2,...
PPX3,...
PPX4,...
RBX1,...
RBX2,...
RBX3,...
RCX1,...
REX1,...
REX2,...
RHX1,...
QSX1,...% overturning
QSX2,...
QSX3,...
QSX4,...
QSX5,...
QSX6,...
QSX7,...
QSX8,...
QSX9,...
QSX10,...
QSX11,...
PPMX1,...
PCY1,...% lateral
PDY1,...
PDY2,...
PDY3,...
PEY1,...
PEY2,...
PEY3,...
PEY4,...
PEY5,...
PKY1,...
PKY2,...
PKY3,...
PKY4,...
PKY5,...
PKY6,...
PKY7,...
PHY1,...
PHY2,...
PVY1,...
PVY2,...
PVY3,...
PVY4,...
PPY1,...
PPY2,...
PPY3,...
PPY4,...
PPY5,...
RBY1,...
RBY2,...
RBY3,...
RBY4,...
RCY1,...
REY1,...
REY2,...
RHY1,...
RHY2,...
RVY1,...
RVY2,...
RVY3,...
RVY4,...
RVY5,...
RVY6,...
QSY1,...% rolling
QSY2,...
QSY3,...
QSY4,...
QSY5,...
QSY6,...
QSY7,...
QSY8,...
QBZ1,...
QBZ2,...
QBZ3,...
QBZ4,...
QBZ5,...
QBZ6,...
QBZ9,...
QBZ10,...
QCZ1,...
QDZ1,...
QDZ2,...
QDZ3,...
QDZ4,...
QDZ6,...
QDZ7,...
QDZ8,...
QDZ9,...
QDZ10,...
QDZ11,...
QEZ1,...
QEZ2,...
QEZ3,...
QEZ4,...
QEZ5,...
QHZ1,...
QHZ2,...
QHZ3,...
QHZ4,...
PPZ1,...
PPZ2,...
SSZ1,...
SSZ2,...
SSZ3,...
SSZ4,...
PDXP1,...% turn slip
PDXP2,...
PDXP3,...
PKYP1,...
PDYP1,...
PDYP2,...
PDYP3,...
PDYP4,...
PHYP1,...
PHYP2,...
PHYP3,...
PHYP4,...
PECP1,...
PECP2,...
QDTP1,...
QCRP1,...% aligning moment
QCRP2,...
QBRP1,...
QDRP1,...
QDRP2,...
WIDTH,...
Q_RA1,... % contact patch
Q_RA2,...
Q_RB1,...
Q_RB2,...
QSX12,...
QSX13,...
QSX14,...
Q_FZ3,...
LONGITUDINAL_STIFFNESS,...% structural
LATERAL_STIFFNESS,...
PCFX1,...
PCFX2,...
PCFX3,...
PCFY1,...
PCFY2,...
PCFY3,...
Fx_ext,...
Fy_ext)
%#codegen
coder.allowpcode('plain')
[Fx,Fy,Fz,Mx,My,Mz,Re,kappa,alpha,sig_x,sig_y,patch_a,patch_b] = vdyncsmtire(omega,Vx,Vy,psidot,gamma,press,scaleFactors,rhoz,plySteer,...
PRESMAX,...
PRESMIN,...
FZMAX,...
FZMIN,...
VXLOW,...
KPUMAX,...
KPUMIN,...
ALPMAX,...
ALPMIN,...
CAMMIN,...
CAMMAX,...
LONGVL,...
UNLOADED_RADIUS,...
NOMPRES,...
FNOMIN,...
VERTICAL_STIFFNESS,...% vertical
DREFF,...
BREFF,...
FREFF,...
Q_RE0,...
Q_V1,...
Q_V2,...
Q_FZ1,...
Q_FZ2,...
Q_FCX,...
Q_FCY,...
PFZ1,...
Q_FCY2,...
PCX1,...% longitudinal
PDX1,...
PDX2,...
PDX3,...
PEX1,...
PEX2,...
PEX3,...
PEX4,...
PKX1,...
PKX2,...
PKX3,...
PHX1,...
PHX2,...
PVX1,...
PVX2,...
PPX1,...
PPX2,...
PPX3,...
PPX4,...
RBX1,...
RBX2,...
RBX3,...
RCX1,...
REX1,...
REX2,...
RHX1,...
QSX1,...% overturning
QSX2,...
QSX3,...
QSX4,...
QSX5,...
QSX6,...
QSX7,...
QSX8,...
QSX9,...
QSX10,...
QSX11,...
PPMX1,...
PCY1,...% lateral
PDY1,...
PDY2,...
PDY3,...
PEY1,...
PEY2,...
PEY3,...
PEY4,...
PEY5,...
PKY1,...
PKY2,...
PKY3,...
PKY4,...
PKY5,...
PKY6,...
PKY7,...
PHY1,...
PHY2,...
PVY1,...
PVY2,...
PVY3,...
PVY4,...
PPY1,...
PPY2,...
PPY3,...
PPY4,...
PPY5,...
RBY1,...
RBY2,...
RBY3,...
RBY4,...
RCY1,...
REY1,...
REY2,...
RHY1,...
RHY2,...
RVY1,...
RVY2,...
RVY3,...
RVY4,...
RVY5,...
RVY6,...
QSY1,...% rolling
QSY2,...
QSY3,...
QSY4,...
QSY5,...
QSY6,...
QSY7,...
QSY8,...
QBZ1,...
QBZ2,...
QBZ3,...
QBZ4,...
QBZ5,...
QBZ6,...
QBZ9,...
QBZ10,...
QCZ1,...
QDZ1,...
QDZ2,...
QDZ3,...
QDZ4,...
QDZ6,...
QDZ7,...
QDZ8,...
QDZ9,...
QDZ10,...
QDZ11,...
QEZ1,...
QEZ2,...
QEZ3,...
QEZ4,...
QEZ5,...
QHZ1,...
QHZ2,...
QHZ3,...
QHZ4,...
PPZ1,...
PPZ2,...
SSZ1,...
SSZ2,...
SSZ3,...
SSZ4,...
PDXP1,...% turn slip
PDXP2,...
PDXP3,...
PKYP1,...
PDYP1,...
PDYP2,...
PDYP3,...
PDYP4,...
PHYP1,...
PHYP2,...
PHYP3,...
PHYP4,...
PECP1,...
PECP2,...
QDTP1,...
QCRP1,...% aligning moment
QCRP2,...
QBRP1,...
QDRP1,...
QDRP2,...
WIDTH,...
Q_RA1,... % contact patch
Q_RA2,...
Q_RB1,...
Q_RB2,...
QSX12,...
QSX13,...
QSX14,...
Q_FZ3,...
LONGITUDINAL_STIFFNESS,...% structural
LATERAL_STIFFNESS,...
PCFX1,...
PCFX2,...
PCFX3,...
PCFY1,...
PCFY2,...
PCFY3,...
Fx_ext,...
Fy_ext);
end

== matlab function vehdynlibtirecommon_TUM/Wheel Module/Brakes/Drum Brake/Drum Brake/Drum Brake Torque Calculation ==
  data: P input; Ba input; T output; mu input; a input; c input; r input; theta1 input; theta2 input
function T=CalcDrumShoeTorque(P,Ba,mu,a,c,r,theta1,theta2)

   %Convert angles from deg to rad
   theta1=theta1*pi/180.;
   theta2=theta2*pi/180.;
     
   %Calculate torque terms
   sigma=cos(theta2)-cos(theta1);
   
   Numerator=pi*mu*c*r*sigma*Ba^2;
   
   Denominator1=2*mu*(-2*r*sigma-a*(cos(theta1)^2-cos(theta2)^2));

   Denominator2=a*(2*theta1-2*theta2-sin(2*theta1)+sin(2*theta2));
    
   %Right shoe torque
   Tr=P*Numerator/(Denominator1+Denominator2);
   
   %Left shoe torque
   Tl=P*Numerator/(-Denominator1+Denominator2);

   T=Tr+Tl;
   
end
